simulink model "nmpc_sim_ee"  (R2022a)
settings: Solver=FixedStepAuto  StartTime=0.0  StopTime=10.5  FixedStep=0.1  RelTol=1e-3
values from neighbouring files (symbols this model uses):
  N = n+6    [nmpc_ee.m]    (also in nmpc_ee_2DoF.m; nmpc_ee_6DoF.m)
  ref = struct()    [nmpc_ee_2DoF.m]    (also in nmpc_ee_6DoF.m)
  Tp = 20    [nmpc_ee.m]    (also in nmpc_ee_2DoF.m = 5; nmpc_ee_6DoF.m = 5)
  Ts = 0.1    [nmpc_ee.m]    (also in nmpc_ee_2DoF.m; nmpc_ee_6DoF.m)
libraries: mpclib x1
settings Model: Creator=charl  LastModifiedBy=charl

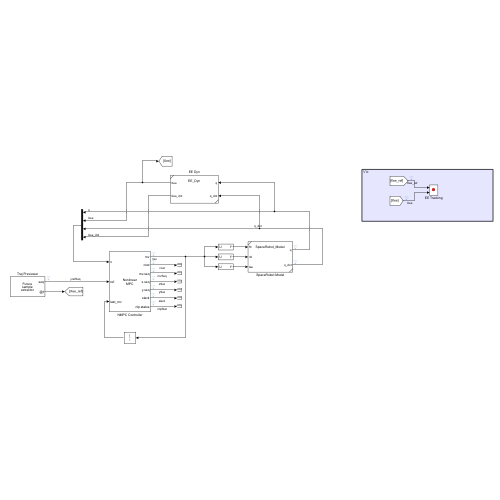
[thumbnail: Simulink's stored preview of the top-level diagram]
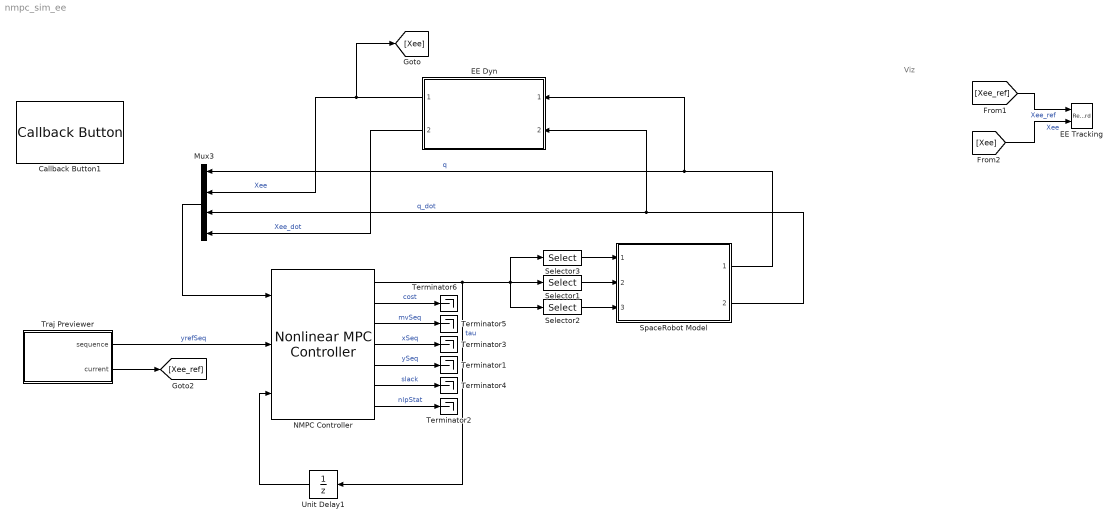
== system nmpc_sim_ee ==
  note: Viz
  Callback Button1 : CallbackButton  ButtonText=Animate results
      settings: ClickFcn=|
      | close all
      | try
      |     sr.animate(out.q, 'fps', 17, 'rate', 1);
      | catch
      |     close all
      | end
  EE Dyn : Subsystem  ReferencedSubsystem=EE_Dyn  spaceRobot=sr
  EE Tracking : Record  FileSettingsInternal="{\"entries\":[{\"content\":{\"excelSettings\":{\"content\":{},\"type\":\"Streamout.ExcelSettings\"}},\"type\":\"Streamout.FileSettingStorage\",\"uuid\":\"963652da-8d4b-469d-8e4c-18dbfe6d1dff\"}],\"packageUris\":[\"http://schema.mathworks.com/mf0/streamout_blocks/R2020a\"],\"version\":\"1.0\"}"  Layout=[1 1]  SignalsInternal="{\"entries\":[{\"content\":{\"signals\":[{\"content\":{\"blockPath\":[\"nmpc_sim_ee/EE Tracking\"],\"channel\":[],\"dimensions\":[3],\"domain\":\"nmpc_sim_ee/EE Tracking\",\"hasChildren\":true,\"lineColor\":\"#7e2f8e\",\"plots\":[],\"port\":1,\"sid\":[],\"signalID\":36,\"signalName\":\"Xee_ref\"},\"type\":\"RecordBlkView.Signal\",\"uuid\":\"22b00cdb-8682-4126-89f8-5e121f10e80f\"},{\"content\":{\"blockPath\":[\"nmpc_sim_ee/EE Tracking\"],\"channel\":[1],\"dimensions\":[3],\"domain\":\"nmpc_sim_ee/EE Tracking\",\"lineColor\":\"#fe330a\",\"parentID\":36,\"plots\":[],\"port\":1,\"sid\":[],\"signalID\":37,\"signalName\":\"Xee_ref\"},\"type\":\"RecordBlkView.Signal\",\"uuid\":\"f790e03b-10c6-4845-8b61-0606bd20cd90\"},{\"content\":{\"blockPath\":[\"nmpc_sim_ee/EE Tracking\"],\"channel\":[2],\"dimensions\":[3],\"domain\":\"nmpc_sim_ee/EE Tracking\",\"lineColor\":\"#64d413\",\"parentID\":36,\"plots\":[],\"port\":1,\"sid\":[],\"signalID\":38,\"signalName\":\"Xee_ref\"},\"type\":\"RecordBlkView.Signal\",\"uuid\":\"ad329607-3211-465a-8a7b-69b199209353\"},{\"content\":{\"blockPath\":[\"nmpc_sim_ee/EE Tracking\"],\"channel\":[3],\"dimensions\":[3],\"domain\":\"nmpc_sim_ee/EE Tracking\",\"lineColor\":\"#ff13a6\",\"parentID\":36,\"plots\":[],\"port\":1,\"sid\":[],\"signalID\":39,\"signalName\":\"Xee_ref\"},\"type\":\"RecordBlkView.Signal\",\"uuid\":\"65231665-f5c0-4a66-93a5-ccc141c8ddfe\"},{\"content\":{\"blockPath\":[\"nmpc_sim_ee/EE Tracking\"],\"channel\":[],\"dimensions\":[6,1],\"domain\":\"nmpc_sim_ee/EE Tracking\",\"hasChildren\":true,\"lineColor\":\"#4dbeee\",\"plots\":[],\"port\":2,\"sid\":[],\"signalID\":45,\"signalName\":\"Xee\"},\"type\":\"RecordBlkView.Signal\",\"uuid\":\"782c644c-a3cd-4b6e-9ef8-35021c75d4d7\"},{\"content\":{\"blockPath\":[\"nmpc_sim_ee/EE Tracking\"],\"channel\":[1,1],\"dimensions\":[6,1],\"domain\":\"nmpc_sim_ee/EE Tracking\",\"lineColor\":\"#0072bd\",\"parentID\":45,\"plots\":[],\"port\":2,\"sid\":[],\"signalID\":46,\"signalName\":\"Xee\"},\"type\":\"RecordBlkView.Signal\",\"uuid\":\"939126b0-8e52-4cd4-b793-9649e04213e8\"},{\"content\":{\"blockPath\":[\"nmpc_sim_ee/EE Tracking\"],\"channel\":[2,1],\"dimensions\":[6,1],\"domain\":\"nmpc_sim_ee/EE Tracking\",\"lineColor\":\"#ff13a6\",\"parentID\":45,\"plots\":[],\"port\":2,\"sid\":[],\"signalID\":47,\"signalName\":\"Xee\"},\"type\":\"RecordBlkView.Signal\",\"uuid\":\"e3b1ee85-709a-4fcc-8d24-b724dc127f8c\"},{\"content\":{\"blockPath\":[\"nmpc_sim_ee/EE Tracking\"],\"channel\":[3,1],\"dimensions\":[6,1],\"domain\":\"nmpc_sim_ee/EE Tracking\",\"lineColor\":\"#fe330a\",\"parentID\":45,\"plots\":[],\"port\":2,\"sid\":[],\"signalID\":48,\"signalName\":\"Xee\"},\"type\":\"RecordBlkView.Signal\",\"uuid\":\"415c915f-dce6-4b91-ba63-ddb1ece5c202\"},{\"content\":{\"blockPath\":[\"nmpc_sim_ee/EE Tracking\"],\"channel\":[4,1],\"dimensions\":[6,1],\"domain\":\"nmpc_sim_ee/EE Tracking\",\"lineColor\":\"#22b573\",\"parentID\":45,\"plots\":[],\"port\":2,\"sid\":[],\"signalID\":49,\"signalName\":\"Xee\"},\"type\":\"RecordBlkView.Signal\",\"uuid\":\"80797cde-a8cd-451d-980f-a0e67f885889\"},{\"content\":{\"blockPath\":[\"nmpc_sim_ee/EE Tracking\"],\"channel\":[5,1],\"dimensions\":[6,1],\"domain\":\"nmpc_sim_ee/EE Tracking\",\"lineColor\":\"#0072bd\",\"parentID\":45,\"plots\":[],\"port\":2,\"sid\":[],\"signalID\":50,\"signalName\":\"Xee\"},\"type\":\"RecordBlkView.Signal\",\"uuid\":\"2c73e0e6-b842-4491-871d-2b2b335ff06d\"},{\"content\":{\"blockPath\":[\"nmpc_sim_ee/EE Tracking\"],\"channel\":[6,1],\"dimensions\":[6,1],\"domain\":\"nmpc_sim_ee/EE Tracking\",\"lineColor\":\"#d95319\",\"parentID\":45,\"plots\":[],\"port\":2,\"sid\":[],\"signalID\":51,\"signalName\":\"Xee\"},\"type\":\"RecordBlkView.Signal\",\"uuid\":\"fcdf8177-5a03-40e3-905a-713274a47c63\"}]},\"type\":\"RecordBlkView.InputSignals\",\"uuid\":\"c6fdc812-1181-43ae-b59d-b621851f7c94\"}],\"packageUris\":[\"http://schema.mathworks.com/mf0/streamout_blocks/R2020a\"],\"version\":\"1.0\"}"  VisualizationBindings="{\"xyplotplugin\":{\"info\":[{\"series\":[],\"subplotID\":1}]}}"  CompatibilityTag=XY
  Mux3 : Mux
  NMPC Controller : mpclib/Nonlinear MPC Controller  SCDEnableBlockLinearizationSpecification=on  nlmpcobj=nlmpc_ee  UseObjectTs=on  TsControl=Ts  UseMEX=off  mexname=nlmpc_ee_SR6_mex  md_enabled=off  mvtarget_enabled=off  param_enabled=off  cost_enabled=on  mvseq_enabled=on  stateseq_enabled=on  ovseq_enabled=on  slack_enabled=on  status_enabled=on  ov_min=off  ov_max=off  mv_min=off  mv_max=off  mvrate_min=off  mvrate_max=off  state_min=off  state_max=off  ov_weight=off  mv_weight=off  mvrate_weight=off  ecr_weight=off  nlp_initialize=off
  Selector1 : Selector  IndexOptions=Index vector (dialog)  Indices=[4:6]  OutputSizes=1
  Selector2 : Selector  IndexOptions=Index vector (dialog)  Indices=[7:N]  OutputSizes=1
  Selector3 : Selector  IndexOptions=Index vector (dialog)  Indices=[1:3]  OutputSizes=1
  SpaceRobot Model : Subsystem  ReferencedSubsystem=SpaceRobot_Model  spaceRobot=sr  jointCstr=off  q_0=q0  q_dot_0=q_dot_0
  Terminator{1..6} (6 alike) : Terminator
  Traj Previewer : Subsystem  mask{signal=ref, ts=Ts, steps=Tp}
      mask prompts: signal "Signal name"; ts "Sampling time"; steps "Number of previewing steps"
      mask init:
      | ts = evalin('base',get_param(gcbh,'ts'));
      | signal = evalin('base',get_param(gcbh,'signal'));
      | steps = evalin('base',get_param(gcbh,'steps'));
      | data = mpc_previewer_maskinit(signal,ts);
      mask Display:
      | fprintf('Future\nsample\nextractor');
      | port_label('output', 1, 'seq')
      | port_label('output', 2, '@t')
  Unit Delay1 : UnitDelay  SampleTime=-1  HasFrameUpgradeWarning=on
  wires:
  NMPC Controller/1 -> Unit Delay1/1, Selector2/1, Selector1/1, Selector3/1  "tau"
  Selector2/1 -> SpaceRobot Model/3
  Selector1/1 -> SpaceRobot Model/2
  Selector3/1 -> SpaceRobot Model/1
  Unit Delay1/1 -> NMPC Controller/3
  Traj Previewer/1(sequence) -> NMPC Controller/2  "yrefSeq"
  SpaceRobot Model/2 -> EE Dyn/2, Mux3/3  "q_dot"
  SpaceRobot Model/1 -> EE Dyn/1, Mux3/1  "q"
  [Xee_ref] -> EE Tracking/1  "Xee_ref"
  [Xee] -> EE Tracking/2  "Xee"
  Mux3/1 -> NMPC Controller/1
  EE Dyn/1 -> [Xee], Mux3/2  "Xee"
  EE Dyn/2 -> Mux3/4  "Xee_dot"
  NMPC Controller/4 -> Terminator3/1  "xSeq"
  NMPC Controller/5 -> Terminator1/1  "ySeq"
  NMPC Controller/7 -> Terminator2/1  "nlpStat"
  Traj Previewer/2(current) -> [Xee_ref]
  NMPC Controller/6 -> Terminator4/1  "slack"
  NMPC Controller/2 -> Terminator6/1  "cost"
  NMPC Controller/3 -> Terminator5/1  "mvSeq"

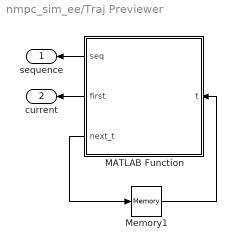
== system nmpc_sim_ee/Traj Previewer ==
  MATLAB Function : MATLAB Function  TreatAsAtomicUnit=on
  Memory1 : Memory  InheritSampleTime=on  LinearizeAsDelay=on
  sequence : Outport
  current : Outport  Port=2
  wires:
  MATLAB Function/1(seq) -> sequence/1
  MATLAB Function/2(first) -> current/1
  Memory1/1 -> MATLAB Function/1(t)
  MATLAB Function/3(next_t) -> Memory1/1

== matlab function nmpc_sim_ee/Traj Previewer/MATLAB Function ==
  settings: updateMethod=DISCRETE  sampleTime=ts
  data: data parameter; seq output; steps parameter; t input; first output; next_t output
function [seq,first,next_t] = fcn(data,steps,t)
%#codegen
[seq,first,next_t] = mpcblock_preview('ref',data,steps,t);
